simulink model "resize_vid"  (R2017a)
settings: Solver=VariableStepAuto  StartTime=0.0  StopTime=inf  RelTol=1e-3
values from neighbouring files (symbols this model uses):
  challenge = [181 165 172 173 159 156 146 161 147 144 154 162 ... (2790525 elements, 725x1283x3)]    [matlab.mat]
libraries: dspvision x2, visiongeotforms x2
settings Model: Creator=ChiChaChai  LastModifiedBy=ChiChaChai

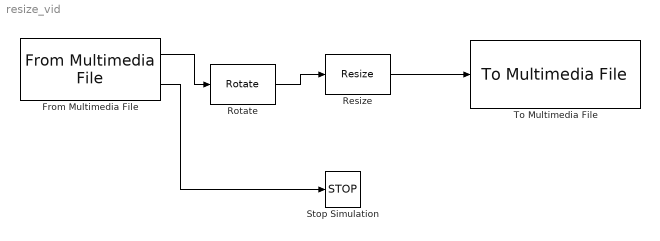
== system resize_vid ==
  From Multimedia File : dspvision/From Multimedia File  inputFilename=C:\Users\ChiChaChai\Documents\AMAS-2017\SelfDrivingCar_with_MATLAB\challenge.mp4  loop=on  numPlays=inf  outputStreams=Video only  videoDataType=single  audioDataType=int16  inheritSampleTime=off  userDefinedSampleTime=1/30  noAudioOutput=off  isIntensityVideo=off  fourcc=RGB  colorVideoFormat=One multidimensional signal  outputEOF=on  dataOrg=Column-major  audioFrameSize=1024  computeAudioFrameSize=off  outSamplingMode=Sample based
      settings: SourceProductBaseCode=VP
  Resize : visiongeotforms/Resize  specify=Number of output rows and columns  rfactor=[200 150]  outCols=25  outRows=25  outRowsCols=[320 240]  interp_method=Bilinear  antialias=on  useROI=off  roiFlag=off  prodOutputMode=Binary point scaling  prodOutputWordLength=32  prodOutputFracLength=10  roundingMode=Nearest  overflowMode=on
      settings: SourceProductName=Computer Vision System Toolbox  SourceProductBaseCode=VP
  Rotate : visiongeotforms/Rotate  outSizeR=Expanded to fit rotated input image  src_angle=Specify via dialog  unit_angle=Degrees  angle=-pi/2  maxAngle=pi  dispImage=Top-left corner  method=Table lookup  fillVal=0  interpMethod=Bilinear  prodOutputMode=Binary point scaling  prodOutputWordLength=32  prodOutputFracLength=10  roundingMode=Nearest  overflowMode=on
      settings: SourceProductName=Computer Vision System Toolbox
  Stop Simulation : Stop
  To Multimedia File : dspvision/To Multimedia File  outputFilename=C:\Users\ChiChaChai\Documents\AMAS-2017\SelfDrivingCar_with_MATLAB\challenge2.mp4  streamSelection=Video only  videoCompressor=None (uncompressed)  audioCompressor=None (uncompressed)  imagePorts=One multidimensional signal  fileType=MPEG4  audioDatatype=Determine from input data type  fourcc=RGB  videoQuality=75  mj2000CompFactor=10
      settings: SourceProductName=Computer Vision System Toolbox  SourceProductBaseCode=VP
  wires:
  From Multimedia File/1 -> Rotate/1
  Resize/1 -> To Multimedia File/1
  From Multimedia File/2 -> Stop Simulation/1
  Rotate/1 -> Resize/1
